simulink model "PLL"  (R2025a)
settings: Solver=FixedStepAuto  StartTime=0.0  StopTime=10.0  FixedStep=Ts  RelTol=1e-3
model mask{GridFrequency=GridFrequency, KiPLLController=KiPLLController, KpPLLController=KpPLLController}
  mask prompts: GridFrequency "Reference Frequency"; KiPLLController "Proportional Gain"; KpPLLController "Integral Gain"
model workspace (MAT data in the model file):
  GridFrequency = 60
  KiPLLController = 0
  KpPLLController = 0
  Ts1 = Simulink.Parameter
  Ts1.Value = 0.001
  Ts1.Complexity = 'real'
  Ts1.Dimensions = [1 1]
  Ts1.DataType = 'auto'
libraries: eeSinusoidalMeasurement x2, simulink x2
settings Model: ParameterArgumentNames=GridFrequency,KiPLLController,KpPLLController  Creator=skota  LastModifiedBy=skota
settings DataIOCC: SaveFormat=StructureWithTime  SaveOutput=off  SignalLogging=off  DSMLogging=off  SaveTime=off  ReturnWorkspaceOutputs=off
settings RTWCC: Toolchain=MinGW64 | CMake/gmake (64-bit Windows)  BuildConfiguration=Release  GPUComputeCapability=3.5

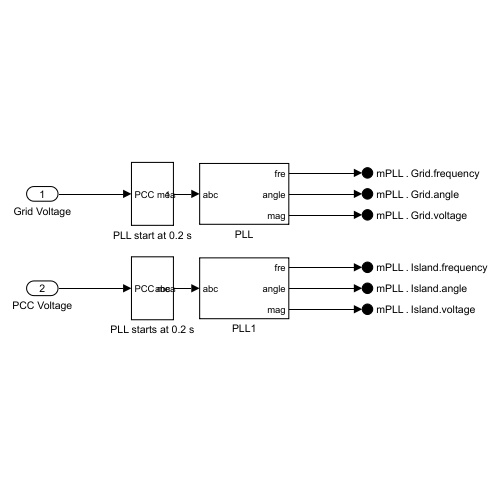
[thumbnail: Simulink's stored preview of the top-level diagram]
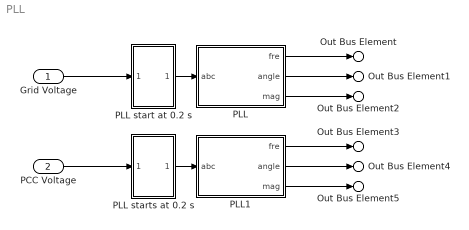
== system PLL ==
  Grid Voltage : Inport
  PCC Voltage : Inport  Port=2
  PLL : Subsystem
  PLL start at 0.2 s : Subsystem
  PLL starts at 0.2 s : Subsystem
  PLL1 : Subsystem
  Out Bus Element : Outport  PortName=mPLL  Element=Grid.frequency
  Out Bus Element1 : Outport  PortName=mPLL  Element=Grid.angle
  Out Bus Element2 : Outport  PortName=mPLL  Element=Grid.voltage
  Out Bus Element3 : Outport  PortName=mPLL  Element=Island.frequency
  Out Bus Element4 : Outport  PortName=mPLL  Element=Island.angle
  Out Bus Element5 : Outport  PortName=mPLL  Element=Island.voltage
  wires:
  PLL/3(mag) -> Out Bus Element2/1
  PLL/1(fre) -> Out Bus Element/1
  PLL start at 0.2 s/1(Out1) -> PLL/1(abc)
  PLL1/3(mag) -> Out Bus Element5/1
  PCC Voltage/1 -> PLL starts at 0.2 s/1(PCC measurement)
  PLL1/2(angle) -> Out Bus Element4/1
  PLL1/1(fre) -> Out Bus Element3/1
  PLL starts at 0.2 s/1(abc) -> PLL1/1(abc)
  Grid Voltage/1 -> PLL start at 0.2 s/1(PCC measurement)
  PLL/2(angle) -> Out Bus Element1/1

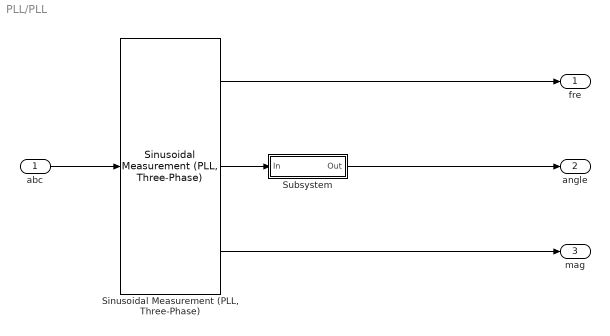
== system PLL/PLL ==
  abc : Inport
  "Sinusoidal Measurement (PLL, Three-Phase)" : eeSinusoidalMeasurement/Sinusoidal Measurement (PLL, Three-Phase)  Kp_LF=KpPLLController  Ki_LF=KiPLLController  F0=GridFrequency  Theta0=0  Ts=Ts1
  Subsystem : Subsystem
  fre : Outport
  angle : Outport  Port=2
  mag : Outport  Port=3
  wires:
  abc/1 -> "Sinusoidal Measurement (PLL, Three-Phase)"/1
  "Sinusoidal Measurement (PLL, Three-Phase)"/3 -> mag/1
  "Sinusoidal Measurement (PLL, Three-Phase)"/2 -> Subsystem/1(In)
  Subsystem/1(Out) -> angle/1
  "Sinusoidal Measurement (PLL, Three-Phase)"/1 -> fre/1

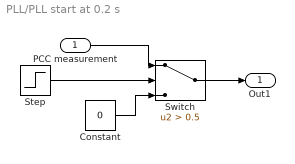
== system PLL/PLL start at 0.2 s ==
  PCC measurement : Inport
  Constant : Constant  Value=0
  Step : Step  Time=0.2  SampleTime=Ts1
  Switch : Switch  Criteria=u2 > Threshold  Threshold=0.5  SaturateOnIntegerOverflow=off  InputSameDT=off
  Out1 : Outport
  wires:
  PCC measurement/1 -> Switch/1
  Switch/1 -> Out1/1
  Constant/1 -> Switch/3
  Step/1 -> Switch/2

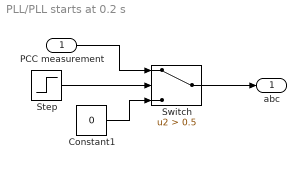
== system PLL/PLL starts at 0.2 s ==
  PCC measurement : Inport
  Constant1 : Constant  Value=0
  Step : Step  Time=0.2  SampleTime=Ts1
  Switch : Switch  Criteria=u2 > Threshold  Threshold=0.5  SaturateOnIntegerOverflow=off  InputSameDT=off
  abc : Outport
  wires:
  PCC measurement/1 -> Switch/1
  Constant1/1 -> Switch/3
  Switch/1 -> abc/1
  Step/1 -> Switch/2

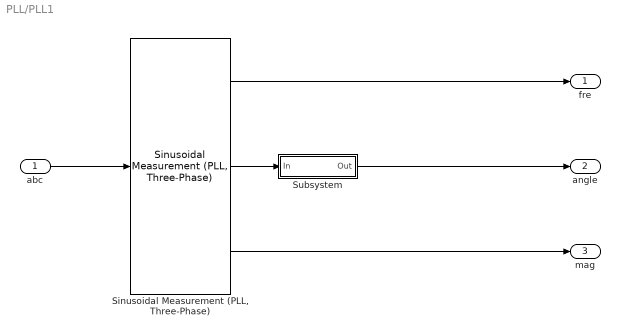
== system PLL/PLL1 ==
  abc : Inport
  "Sinusoidal Measurement (PLL, Three-Phase)" : eeSinusoidalMeasurement/Sinusoidal Measurement (PLL, Three-Phase)  Kp_LF=KpPLLController  Ki_LF=KiPLLController  F0=GridFrequency  Theta0=0  Ts=Ts1
  Subsystem : Subsystem
  fre : Outport
  angle : Outport  Port=2
  mag : Outport  Port=3
  wires:
  "Sinusoidal Measurement (PLL, Three-Phase)"/1 -> fre/1
  Subsystem/1(Out) -> angle/1
  "Sinusoidal Measurement (PLL, Three-Phase)"/2 -> Subsystem/1(In)
  "Sinusoidal Measurement (PLL, Three-Phase)"/3 -> mag/1
  abc/1 -> "Sinusoidal Measurement (PLL, Three-Phase)"/1

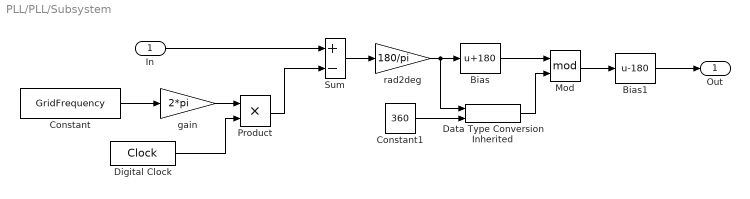
== system PLL/PLL/Subsystem ==
  In : Inport
  Bias : Bias  Bias=180  SaturateOnIntegerOverflow=off
  Bias1 : Bias  Bias=-180  SaturateOnIntegerOverflow=off
  Constant : Constant  Value=GridFrequency
  Constant1 : Constant  Value=360
  Data Type Conversion Inherited : simulink/Signal Attributes/Data Type Conversion Inherited  ConvertRealWorld=Real World Value  DoSatur=off
  Digital Clock : DigitalClock  SampleTime=Ts1
  Mod : Math  Operator=mod
  Product : Product
  Sum : Sum  Inputs=+-  OutDataTypeStr=Inherit: Same as first input
  gain : Gain  Gain=2*pi
  rad2deg : Gain  Gain=180/pi
  Out : Outport
  wires:
  Data Type Conversion Inherited/1 -> Mod/2
  Sum/1 -> rad2deg/1
  rad2deg/1 -> Bias/1, Data Type Conversion Inherited/1
  Constant1/1 -> Data Type Conversion Inherited/2
  Digital Clock/1 -> Product/2
  Mod/1 -> Bias1/1
  Bias/1 -> Mod/1
  Constant/1 -> gain/1
  gain/1 -> Product/1
  In/1 -> Sum/1
  Product/1 -> Sum/2
  Bias1/1 -> Out/1

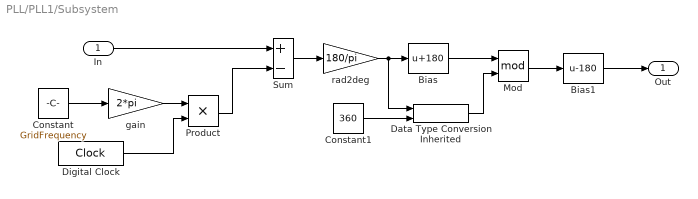
== system PLL/PLL1/Subsystem ==
  In : Inport
  Bias : Bias  Bias=180  SaturateOnIntegerOverflow=off
  Bias1 : Bias  Bias=-180  SaturateOnIntegerOverflow=off
  Constant : Constant  Value=GridFrequency
  Constant1 : Constant  Value=360
  Data Type Conversion Inherited : simulink/Signal Attributes/Data Type Conversion Inherited  ConvertRealWorld=Real World Value  DoSatur=off
  Digital Clock : DigitalClock  SampleTime=Ts1
  Mod : Math  Operator=mod
  Product : Product
  Sum : Sum  Inputs=+-  OutDataTypeStr=Inherit: Same as first input
  gain : Gain  Gain=2*pi
  rad2deg : Gain  Gain=180/pi
  Out : Outport
  wires:
  Bias1/1 -> Out/1
  Product/1 -> Sum/2
  In/1 -> Sum/1
  gain/1 -> Product/1
  Constant/1 -> gain/1
  Bias/1 -> Mod/1
  Mod/1 -> Bias1/1
  Digital Clock/1 -> Product/2
  Constant1/1 -> Data Type Conversion Inherited/2
  rad2deg/1 -> Data Type Conversion Inherited/1, Bias/1
  Sum/1 -> rad2deg/1
  Data Type Conversion Inherited/1 -> Mod/2
